simulink model "ModelMotS_AlphaBeta_bis_FVC"  (R2018b)
settings: Solver=ode45  StartTime=0.0  StopTime=1200  MaxStep=1e-4  RelTol=1e-4  EnableMultiTasking=on
values from neighbouring files (symbols this model uses):
  Data_Ts = 0.005    [gen_sim_alpha_beta.m]    (also in gen_sim_dq.m = 0.00025)
  Inom = 9.1    [gen_sim_alpha_beta.m]    (also in gen_sim_dq.m)
  J = 0.045    [gen_sim_alpha_beta.m]    (also in gen_sim_dq.m; gen_sim_new_data_december.m)
  Jm = J    (= 0.045)    [gen_sim_alpha_beta.m]    (also in gen_sim_dq.m)
  Lfr = 0.007    [gen_sim_alpha_beta.m]    (also in gen_sim_dq.m; gen_sim_new_data_december.m)
  Lfs = 0.007    [gen_sim_alpha_beta.m]    (also in gen_sim_dq.m; gen_sim_new_data_december.m)
  Lm = 0.153    [gen_sim_alpha_beta.m]    (also in gen_sim_dq.m; gen_sim_new_data_december.m)
  Lmt = 0.210    (= 0.21)    [gen_sim_alpha_beta.m]    (also in gen_sim_dq.m; gen_sim_new_data_december.m)
  Lr = 0.160    (= 0.16)    [gen_sim_alpha_beta.m]    (also in gen_sim_dq.m; gen_sim_new_data_december.m)
  Ls = 0.160    (= 0.16)    [gen_sim_alpha_beta.m]    (also in gen_sim_dq.m; gen_sim_new_data_december.m)
  np = 2    [gen_sim_alpha_beta.m]    (also in gen_sim_dq.m; gen_sim_new_data_december.m)
  P1 = 0.7    [gen_sim_alpha_beta.m]    (also in gen_sim_dq.m; gen_sim_new_data_december.m)
  P2 = 1.5    [gen_sim_alpha_beta.m]    (also in gen_sim_dq.m; gen_sim_new_data_december.m)
  Prdnom = 1    [gen_sim_alpha_beta.m]    (also in gen_sim_dq.m)
  Prinit = [ 0 ; 0 ]    [gen_sim_alpha_beta.m]    (also in gen_sim_dq.m; gen_sim_new_data_december.m)
  Psinit = [ 0 ; 0 ]    [gen_sim_alpha_beta.m]    (also in gen_sim_dq.m; gen_sim_new_data_december.m)
  Rr = 0.9    [gen_sim_alpha_beta.m]    (also in gen_sim_dq.m; gen_sim_new_data_december.m)
  Rs = 1.5    [gen_sim_alpha_beta.m]    (also in gen_sim_dq.m; gen_sim_new_data_december.m)
  SFC_Coeff = 100    [gen_sim_alpha_beta.m]    (also in gen_sim_dq.m)
  SLP_Coeff = 100    [gen_sim_alpha_beta.m]    (also in gen_sim_dq.m)
  Speed = data.speed_true    [Plot_EncoderDecoder_Output.m]    (also in TreatModelMot_dq.m = Data.Speed.Data / (2*pi); test1.mat = [0 0 0 0 0 0 0 0 0 0 0 0 ... (601 elements, 601x1)]; test2.mat = [0 0 0 0 0 0 0 0 0 0 0 0 ... (601 elements, 601x1)])
  thrinit = 0    [gen_sim_alpha_beta.m]    (also in gen_sim_dq.m; gen_sim_new_data_december.m)
  Tn = 25    [gen_sim_alpha_beta.m]    (also in gen_sim_dq.m; gen_sim_new_data_december.m)
  Tpwm = Ts    (= 0.00025)    [gen_sim_alpha_beta.m]    (also in gen_sim_dq.m)
  Vnom = 400    [gen_sim_alpha_beta.m]    (also in gen_sim_dq.m)
  wCurr = 0    [gen_sim_alpha_beta.m]    (also in gen_sim_dq.m)
  wCurr_PI = 2*pi*50    (= 314.159265359)    [gen_sim_alpha_beta.m]    (also in gen_sim_dq.m)
  wL = 2*pi*0    (= 0)    [gen_sim_alpha_beta.m]    (also in gen_sim_dq.m; gen_sim_new_data_december.m)
  wn = 2*pi*50    (= 314.159265359)    [gen_sim_alpha_beta.m]    (also in gen_sim_dq.m; gen_sim_new_data_december.m)
  wrinit = 2*pi*0    (= 0)    [gen_sim_alpha_beta.m]    (also in gen_sim_dq.m; gen_sim_new_data_december.m)
  wSpeed_PI = 2*pi*2.5    (= 15.7079632679)    [gen_sim_alpha_beta.m]    (also in gen_sim_dq.m)
  wSpeedEst = 2*pi*500    (= 3141.59265359)    [gen_sim_alpha_beta.m]    (also in gen_sim_dq.m)
  xiCurr_PI = 1/2    (= 0.5)    [gen_sim_alpha_beta.m]    (also in gen_sim_dq.m)
  xiSpeed_PI = 1    [gen_sim_alpha_beta.m]    (also in gen_sim_dq.m)
undefined symbols (not defined in the file or in its folder): DiscIntNeverNeededParam, TorqueLoad
libraries: simulink x7
settings Model: Creator=stbp106  LastModifiedBy=SESA336393
settings DataIOCC: LimitDataPoints=on  SaveFormat=Array
settings OptimizationCC: LifeSpan=inf
settings DebuggingCC: UnderspecifiedInitializationDetection=Classic  MergeDetectMultiDrivingBlocksExec=none  SolverPrmCheckMsg=warning  SFUnexpectedBacktrackingDiag=warning  SFNoUnconditionalDefaultTransitionDiag=warning  SFExecutionAtInitializationDiag=none
settings HardwareCC: ProdBitPerPointer=32  ProdBitPerSizeT=32  ProdBitPerPtrDiffT=32  ProdLargestAtomicFloat=None  ProdIntDivRoundTo=Undefined  ProdEndianess=Unspecified  ProdWordSize=32  ProdHWDeviceType=32-bit Generic
settings ModelReferenceCC: PropagateSignalLabelsOutOfModel=off
settings SFSimCC: SimUseLocalCustomCode=off
settings RTWCC: RTWUseLocalCustomCode=off
settings CodeAppCC: StateflowObjectComments=on
settings GRTTargetCC: TargetLangStandard=C89/C90 (ANSI)  GeneratePreprocessorConditionals=Disable all
settings ConfigComp: CovMetricSettings=dw  CovHtmlReporting=on  CovSaveCumulativeToWorkspaceVar=on  CovSaveSingleToWorkspaceVar=on  CovExternalEMLEnable=off  CovSFcnEnable=off

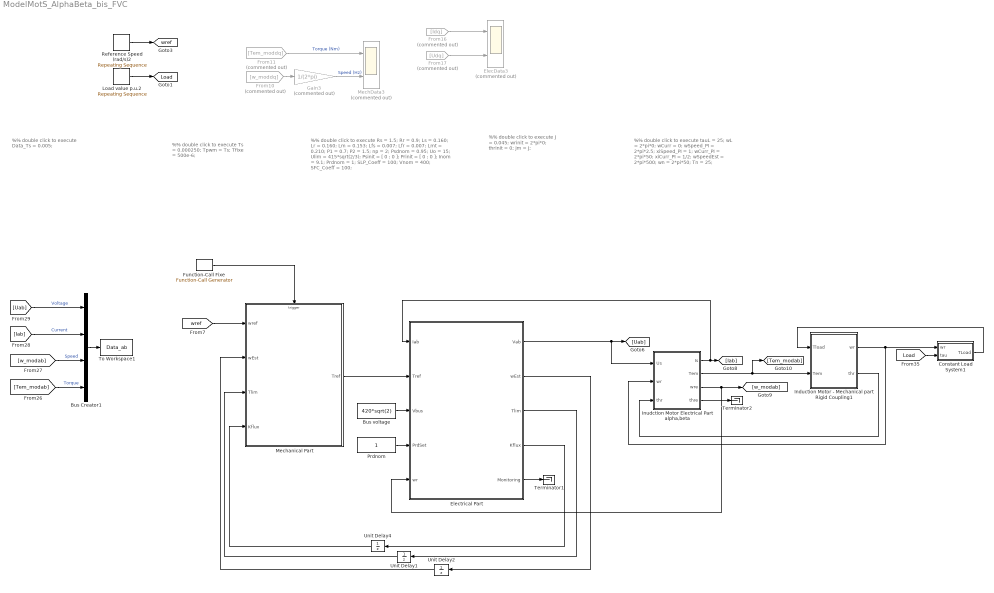
== system ModelMotS_AlphaBeta_bis_FVC ==
  note: %% double click to execute
      |
      | Rs = 1.5; Rr = 0.9;
      | Ls = 0.160; Lr = 0.160; Lm = 0.153;
      | Lfs = 0.007; Lfr = 0.007; Lmt = 0.210; P1 = 0.7; P2 = 1.5;
      | np = 2;
      | Psdnom = 0.95; Uo = 15; Ulim = 415*sqrt(2/3);
      | Psinit = [ 0 ; 0 ]; Prinit = [ 0 ; 0 ];
      | Inom = 9.1; Prdnom = 1; SLP_Coeff = 100; Vnom = 400;
      | SFC_Coeff = 100;
  note: %% double click to execute
      |
      | J = 0.045;
      | wrinit = 2*pi*0;
      | thrinit = 0;
      | Jm = J;
  note: %% double click to execute
      |
      | tauL = 25;
      | wL = 2*pi*0;
      |
      | wCurr = 0;
      | wSpeed_PI = 2*pi*2.5; xiSpeed_PI = 1;
      | wCurr_PI = 2*pi*50; xiCurr_PI = 1/2;
      | wSpeedEst = 2*pi*500;
      |
      | wn = 2*pi*50;
      | Tn = 25;
  note: %% double click to execute
      |
      | Ts = 0.000250;
      | Tpwm = Ts;
      | Tfixe = 500e-6;
  note: %% double click to execute
      |
      | Data_Ts = 0.005;
  Bus Creator1 : BusCreator  Inputs=4
  Bus voltage : Constant  Value=420*sqrt(2)
  Constant Load System1 : Subsystem  Description=""
  ElecData3 : Scope  Commented=on  NumInputPorts=2
  Electrical Part : Subsystem
  From10 : From  Commented=on  GotoTag=w_moddq
  From11 : From  Commented=on  GotoTag=Tem_moddq
  From16 : From  Commented=on  GotoTag=Idq
  From17 : From  Commented=on  GotoTag=Udq
  Function-Call Fixe : simulink/Ports & Subsystems/Function-Call Generator  sample_time=Tfixe  numberOfIterations=1
  Gain3 : Gain  Commented=on  Gain=1/(2*pi)  SaturateOnIntegerOverflow=on  OutDataTypeStr=Inherit: Same as input  ParamDataTypeStr=Inherit: Same as input
  Induction Motor - Mechanical part Rigid Coupling1 : Subsystem  Description=""
  Inudction Motor Electrical Part alpha,beta : Subsystem  Description=""
  Load value p.u.2 : simulink/Sources/Repeating Sequence  rep_seq_t=t  rep_seq_y=TorqueLoad*Tn
  MechData3 : Scope  Commented=on  NumInputPorts=2
  Mechanical Part : Subsystem
  Prdnom : Constant
  Reference Speed (rad/s)2 : simulink/Sources/Repeating Sequence  rep_seq_t=t  rep_seq_y=Speed*wn
  Terminator1 : Terminator
  Terminator2 : Terminator
  To Workspace1 : ToWorkspace  VariableName=Data_ab  SaveFormat=Timeseries  SampleTime=Data_Ts
  Unit Delay1 : UnitDelay  SampleTime=-1
  Unit Delay2 : UnitDelay  SampleTime=-1
  Unit Delay4 : UnitDelay  SampleTime=-1
  tag scope: Load=global, wref=global
  wires:
  From16/1 -> ElecData3/1
  From17/1 -> ElecData3/2
  From10/1 -> Gain3/1
  From11/1 -> MechData3/1  "Torque (Nm)"
  Gain3/1 -> MechData3/2  "Speed (Hz)"
  Induction Motor - Mechanical part Rigid Coupling1/2(thr) -> Inudction Motor Electrical Part alpha,beta/3(thr)
  Inudction Motor Electrical Part alpha,beta/2(Tem) -> [Tem_modab], Induction Motor - Mechanical part Rigid Coupling1/2(Tem)
  Induction Motor - Mechanical part Rigid Coupling1/1(wr) -> Constant Load System1/1(wr), Inudction Motor Electrical Part alpha,beta/2(wr)
  Inudction Motor Electrical Part alpha,beta/4(thre) -> Terminator2/1
  Constant Load System1/1(TLoad) -> Induction Motor - Mechanical part Rigid Coupling1/1(Tload)
  [Load] -> Constant Load System1/2(tau)
  Electrical Part/1(Vab) -> Inudction Motor Electrical Part alpha,beta/1(Us), [Uab]
  Reference Speed (rad/s)2/1 -> [wref]
  Load value p.u.2/1 -> [Load]
  Prdnom/1 -> Electrical Part/4(PrdSet)
  Inudction Motor Electrical Part alpha,beta/3(wre) -> Electrical Part/5(wr), [w_modab]
  Electrical Part/3(Tlim) -> Unit Delay1/1
  Electrical Part/4(Kflux) -> Unit Delay4/1
  Unit Delay1/1 -> Mechanical Part/3(Tlim)
  [wref] -> Mechanical Part/1(wref)
  Unit Delay4/1 -> Mechanical Part/4(Kflux)
  Bus voltage/1 -> Electrical Part/3(Vbus)
  Unit Delay2/1 -> Mechanical Part/2(wEst)
  Mechanical Part/1(Tref) -> Electrical Part/2(Tref)
  Inudction Motor Electrical Part alpha,beta/1(Is) -> Electrical Part/1(Iab), [Iab]
  Function-Call Fixe/1 -> Mechanical Part/Trigger
  Electrical Part/2(wEst) -> Unit Delay2/1
  Electrical Part/5(Monitoring) -> Terminator1/1
  Bus Creator1/1 -> To Workspace1/1
  [w_modab] -> Bus Creator1/3  "Speed"
  [Tem_modab] -> Bus Creator1/4  "Torque"
  [Iab] -> Bus Creator1/2  "Current"
  [Uab] -> Bus Creator1/1  "Voltage"

== system ModelMotS_AlphaBeta_bis_FVC/Constant Load System1 ==
  wr : Inport
  tau : Inport  Port=2
  Constant1 : Constant  Value=wL
  Fcn : Fcn  Expr=u(1)/sqrt( u(1)^2 + (2*pi*0.1)^2)
  Product2 : Product  RndMeth=Zero
  Sum2 : Sum  Inputs=+-  SaturateOnIntegerOverflow=on  InputSameDT=on  OutDataTypeStr=Inherit: Same as first input
  TLoad : Outport
  wires:
  Product2/1 -> TLoad/1
  wr/1 -> Sum2/1
  Constant1/1 -> Sum2/2
  Sum2/1 -> Fcn/1
  Fcn/1 -> Product2/1
  tau/1 -> Product2/2

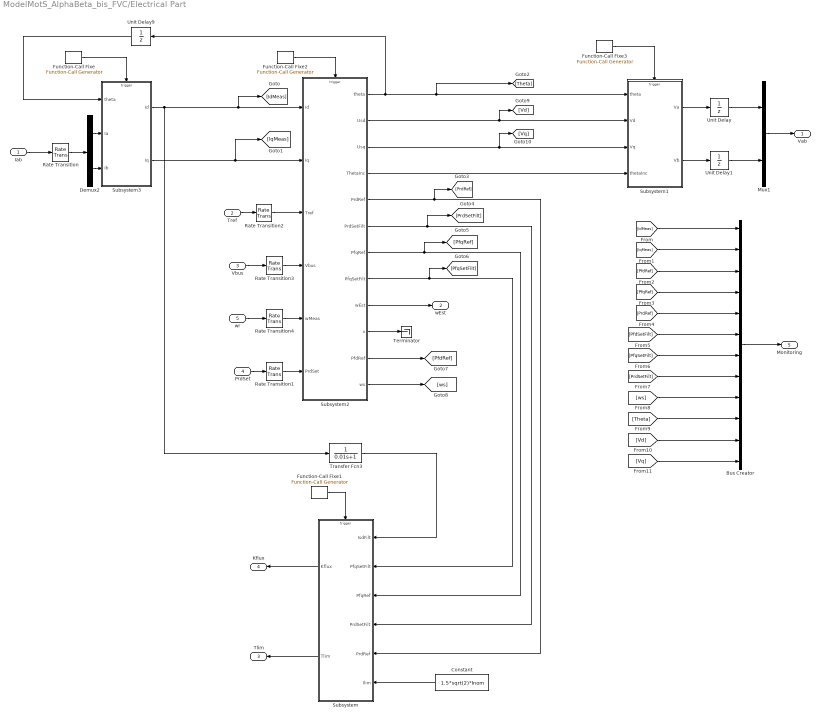
== system ModelMotS_AlphaBeta_bis_FVC/Electrical Part ==
  Iab : Inport
  Tref : Inport  Port=2
  Vbus : Inport  Port=3
  PrdSet : Inport  Port=4
  wr : Inport  Port=5
  Bus Creator : BusCreator  Inputs=12
  Constant : Constant  Value=1.5*sqrt(2)*Inom
  Demux2 : Demux  Outputs=2
  Function-Call Fixe : simulink/Ports & Subsystems/Function-Call Generator  sample_time=Tpwm  numberOfIterations=1
  Function-Call Fixe1 : simulink/Ports & Subsystems/Function-Call Generator  sample_time=Tfixe  numberOfIterations=1
  Function-Call Fixe2 : simulink/Ports & Subsystems/Function-Call Generator  sample_time=Tpwm  numberOfIterations=1
  Function-Call Fixe3 : simulink/Ports & Subsystems/Function-Call Generator  sample_time=Tpwm  numberOfIterations=1
  Mux1 : Mux  Inputs=2
  Rate Transition{,1..4} (5 alike) : RateTransition
  Subsystem : Subsystem
  Subsystem1 : Subsystem
  Subsystem2 : Subsystem
  Subsystem3 : Subsystem
  Terminator : Terminator
  Transfer Fcn3 : TransferFcn  Denominator=[0.01 1]
  Unit Delay : UnitDelay  SampleTime=-1
  Unit Delay1 : UnitDelay  SampleTime=-1
  Unit Delay9 : UnitDelay  SampleTime=-1
  Vab : Outport
  wEst : Outport  Port=2
  Tlim : Outport  Port=3
  Kflux : Outport  Port=4
  Monitoring : Outport  Port=5
  wires:
  [IqMeas] -> Bus Creator/2
  [IdMeas] -> Bus Creator/1
  [PfdRef] -> Bus Creator/3
  [PfqRef] -> Bus Creator/4
  [PrdRef] -> Bus Creator/5
  [PrdSetFilt] -> Bus Creator/8
  [PfqSetFilt] -> Bus Creator/7
  [PfdSetFilt] -> Bus Creator/6
  [ws] -> Bus Creator/9
  [Theta] -> Bus Creator/10
  Bus Creator/1 -> Monitoring/1
  Transfer Fcn3/1 -> Subsystem/1(IsdFilt)
  Subsystem/1(Kflux) -> Kflux/1
  Subsystem/2(Tlim) -> Tlim/1
  Subsystem1/1(Va) -> Unit Delay/1
  [Vd] -> Bus Creator/11
  [Vq] -> Bus Creator/12
  Subsystem2/7(PfqRef) -> [PfqRef], Subsystem/3(PfqRef)
  Subsystem2/6(PrdSetFilt) -> [PrdSetFilt], Subsystem/4(PrdSetFilt)
  Subsystem2/8(PfqSetFilt) -> [PfqSetFilt], Subsystem/2(PfqSetFilt)
  Subsystem2/1(theta) -> Subsystem1/1(theta), [Theta], Unit Delay9/1
  Subsystem2/5(PrdRef) -> [PrdRef], Subsystem/5(PrdRef)
  Subsystem2/3(Usq) -> [Vq], Subsystem1/3(Vq)
  Subsystem2/2(Usd) -> Subsystem1/2(Vd), [Vd]
  Tref/1 -> Rate Transition2/1
  Vbus/1 -> Rate Transition3/1
  wr/1 -> Rate Transition4/1
  Subsystem2/4(ThetaInc) -> Subsystem1/4(thetaInc)
  Subsystem2/9(wEst) -> wEst/1
  Subsystem2/11(PfdRef) -> [PfdRef]
  Subsystem2/12(ws) -> [ws]
  Subsystem3/2(Iq) -> [IqMeas], Subsystem2/2(Iq)
  Subsystem3/1(Id) -> Transfer Fcn3/1, Subsystem2/1(Id), [IdMeas]
  Unit Delay9/1 -> Subsystem3/1(theta)
  Iab/1 -> Rate Transition/1
  Function-Call Fixe/1 -> Subsystem3/Trigger
  Function-Call Fixe2/1 -> Subsystem2/Trigger
  Function-Call Fixe3/1 -> Subsystem1/Trigger
  Function-Call Fixe1/1 -> Subsystem/Trigger
  Rate Transition2/1 -> Subsystem2/3(Tref)
  Subsystem2/10(x) -> Terminator/1
  Constant/1 -> Subsystem/6(Ilim)
  Rate Transition3/1 -> Subsystem2/4(Vbus)
  Rate Transition4/1 -> Subsystem2/5(wMeas)
  Rate Transition/1 -> Demux2/1
  Demux2/1 -> Subsystem3/2(Ia)
  Demux2/2 -> Subsystem3/3(Ib)
  Subsystem1/2(Vb) -> Unit Delay1/1
  Unit Delay/1 -> Mux1/1
  Unit Delay1/1 -> Mux1/2
  Mux1/1 -> Vab/1
  PrdSet/1 -> Rate Transition1/1
  Rate Transition1/1 -> Subsystem2/6(PrdSet)

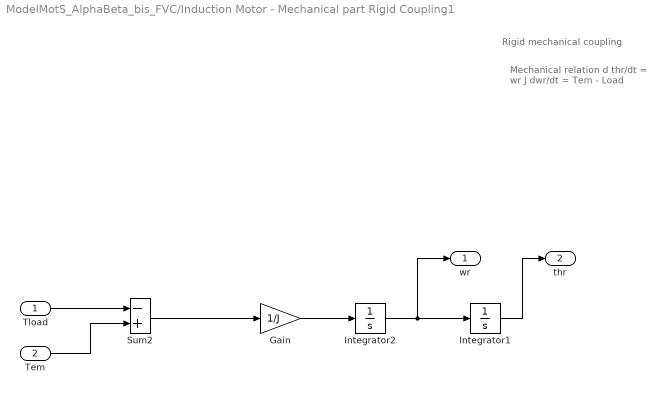
== system ModelMotS_AlphaBeta_bis_FVC/Induction Motor - Mechanical part Rigid Coupling1 ==
  note: Mechanical relation
      | d thr/dt = wr
      | J dwr/dt = Tem - Load
  note: Rigid mechanical coupling
  Tload : Inport
  Tem : Inport  Port=2
  Gain : Gain  Gain=1/J  SaturateOnIntegerOverflow=on  OutDataTypeStr=Inherit: Same as input  ParamDataTypeStr=Inherit: Same as input
  Integrator1 : Integrator  InitialCondition=thrinit
  Integrator2 : Integrator  InitialCondition=wrinit
  Sum2 : Sum  Inputs=-+  SaturateOnIntegerOverflow=on  InputSameDT=on  OutDataTypeStr=Inherit: Same as first input
  wr : Outport
  thr : Outport  Port=2
  wires:
  Sum2/1 -> Gain/1
  Gain/1 -> Integrator2/1
  Tload/1 -> Sum2/1
  Tem/1 -> Sum2/2
  Integrator2/1 -> Integrator1/1, wr/1
  Integrator1/1 -> thr/1

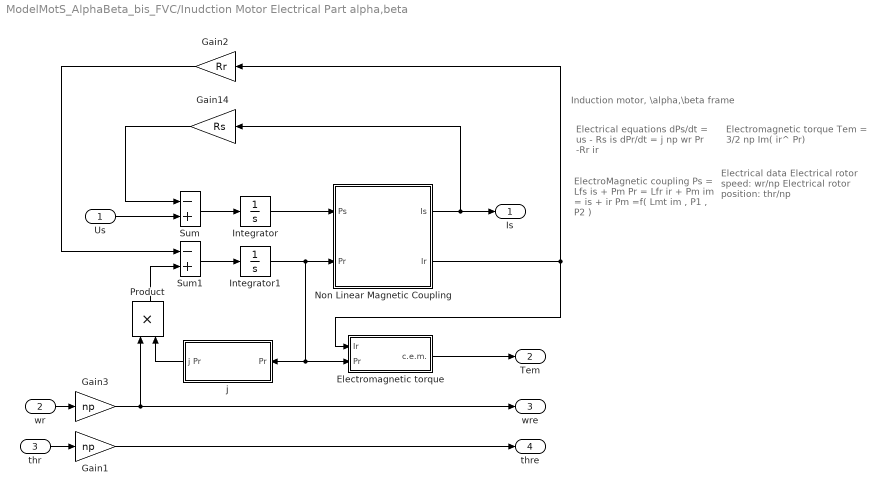
== system ModelMotS_AlphaBeta_bis_FVC/Inudction Motor Electrical Part alpha,beta ==
  note: Electrical equations
      | dPs/dt = us - Rs is
      | dPr/dt = j np wr Pr -Rr ir
  note: ElectroMagnetic coupling
      | Ps  = Lfs is + Pm
      | Pr  = Lfr ir + Pm
      |
      | im = is + ir
      | Pm =f( Lmt im , P1 , P2 )
  note: Electromagnetic torque
      | Tem = 3/2 np Im( ir^ Pr)
  note: Induction motor, \alpha,\beta frame
  note: Electrical data
      | Electrical rotor speed: wr/np
      | Electrical rotor position: thr/np
  Us : Inport
  wr : Inport  Port=2
  thr : Inport  Port=3
  Electromagnetic torque : Subsystem
  Gain1 : Gain  Gain=np  SaturateOnIntegerOverflow=on  OutDataTypeStr=Inherit: Same as input  ParamDataTypeStr=Inherit: Same as input
  Gain14 : Gain  Gain=Rs  SaturateOnIntegerOverflow=on  OutDataTypeStr=Inherit: Same as input  ParamDataTypeStr=Inherit: Same as input
  Gain2 : Gain  Gain=Rr  SaturateOnIntegerOverflow=on  OutDataTypeStr=Inherit: Same as input  ParamDataTypeStr=Inherit: Same as input
  Gain3 : Gain  Gain=np  SaturateOnIntegerOverflow=on  OutDataTypeStr=Inherit: Same as input  ParamDataTypeStr=Inherit: Same as input
  Integrator : Integrator  InitialCondition=Psinit
  Integrator1 : Integrator  InitialCondition=Prinit
  Non Linear Magnetic Coupling : Subsystem
  Product : Product  SaturateOnIntegerOverflow=on  RndMeth=Zero  InputSameDT=on  OutDataTypeStr=Inherit: Same as first input
  Sum : Sum  Inputs=-+  SaturateOnIntegerOverflow=on  InputSameDT=on  OutDataTypeStr=Inherit: Same as first input
  Sum1 : Sum  Inputs=-+  SaturateOnIntegerOverflow=on  InputSameDT=on  OutDataTypeStr=Inherit: Same as first input
  j : Subsystem
  Is : Outport
  Tem : Outport  Port=2
  wre : Outport  Port=3
  thre : Outport  Port=4
  wires:
  Sum/1 -> Integrator/1
  Non Linear Magnetic Coupling/1(Is) -> Gain14/1, Is/1
  Gain14/1 -> Sum/1
  Us/1 -> Sum/2
  Sum1/1 -> Integrator1/1
  Gain2/1 -> Sum1/1
  j/1(j Pr) -> Product/2
  Product/1 -> Sum1/2
  Non Linear Magnetic Coupling/2(Ir) -> Electromagnetic torque/1(Ir), Gain2/1
  Electromagnetic torque/1(c.e.m.) -> Tem/1
  Integrator/1 -> Non Linear Magnetic Coupling/1(Ps)
  Integrator1/1 -> Non Linear Magnetic Coupling/2(Pr), j/1(Pr), Electromagnetic torque/2(Pr)
  Gain3/1 -> Product/1, wre/1
  wr/1 -> Gain3/1
  thr/1 -> Gain1/1
  Gain1/1 -> thre/1

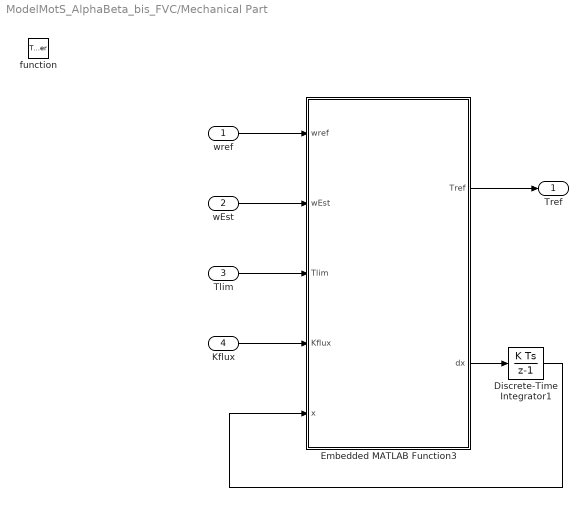
== system ModelMotS_AlphaBeta_bis_FVC/Mechanical Part ==
  wref : Inport
  wEst : Inport  Port=2
  Tlim : Inport  Port=3
  Kflux : Inport  Port=4
  function : TriggerPort  TriggerType=function-call  VariantControl=(inherit)
  Discrete-Time Integrator1 : DiscreteIntegrator  InitialCondition=zeros(1,2)  SampleTime=-1  ICPrevOutput=DiscIntNeverNeededParam  ICPrevScaledInput=DiscIntNeverNeededParam
  Embedded MATLAB Function3 : MATLAB Function  TreatAsAtomicUnit=on
  Tref : Outport
  wires:
  Discrete-Time Integrator1/1 -> Embedded MATLAB Function3/5(x)
  wEst/1 -> Embedded MATLAB Function3/2(wEst)
  Tlim/1 -> Embedded MATLAB Function3/3(Tlim)
  wref/1 -> Embedded MATLAB Function3/1(wref)
  Embedded MATLAB Function3/2(dx) -> Discrete-Time Integrator1/1
  Embedded MATLAB Function3/1(Tref) -> Tref/1
  Kflux/1 -> Embedded MATLAB Function3/4(Kflux)

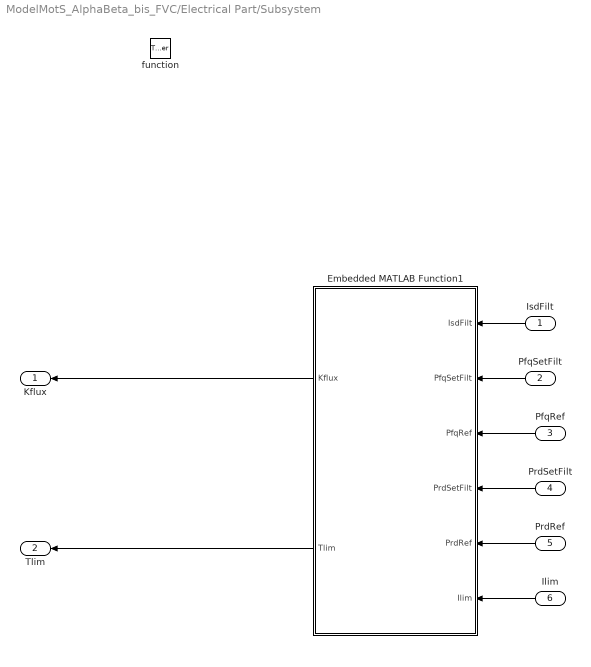
== system ModelMotS_AlphaBeta_bis_FVC/Electrical Part/Subsystem ==
  IsdFilt : Inport
  PfqSetFilt : Inport  Port=2
  PfqRef : Inport  Port=3
  PrdSetFilt : Inport  Port=4
  PrdRef : Inport  Port=5
  Ilim : Inport  Port=6
  function : TriggerPort  TriggerType=function-call  VariantControl=(inherit)
  Embedded MATLAB Function1 : MATLAB Function  TreatAsAtomicUnit=on
  Kflux : Outport
  Tlim : Outport  Port=2
  wires:
  Embedded MATLAB Function1/2(Tlim) -> Tlim/1
  IsdFilt/1 -> Embedded MATLAB Function1/1(IsdFilt)
  Embedded MATLAB Function1/1(Kflux) -> Kflux/1
  PrdSetFilt/1 -> Embedded MATLAB Function1/4(PrdSetFilt)
  PfqSetFilt/1 -> Embedded MATLAB Function1/2(PfqSetFilt)
  PfqRef/1 -> Embedded MATLAB Function1/3(PfqRef)
  PrdRef/1 -> Embedded MATLAB Function1/5(PrdRef)
  Ilim/1 -> Embedded MATLAB Function1/6(Ilim)

== system ModelMotS_AlphaBeta_bis_FVC/Electrical Part/Subsystem1 ==
  theta : Inport
  Vd : Inport  Port=2
  Vq : Inport  Port=3
  thetaInc : Inport  Port=4
  function : TriggerPort  TriggerType=function-call  VariantControl=(inherit)
  Embedded MATLAB Function5 : MATLAB Function  TreatAsAtomicUnit=on
  Va : Outport
  Vb : Outport  Port=2
  wires:
  Embedded MATLAB Function5/1(Va) -> Va/1
  Vd/1 -> Embedded MATLAB Function5/1(Vd)
  thetaInc/1 -> Embedded MATLAB Function5/4(thetaInc)
  Embedded MATLAB Function5/2(Vb) -> Vb/1
  Vq/1 -> Embedded MATLAB Function5/2(Vq)
  theta/1 -> Embedded MATLAB Function5/3(theta)

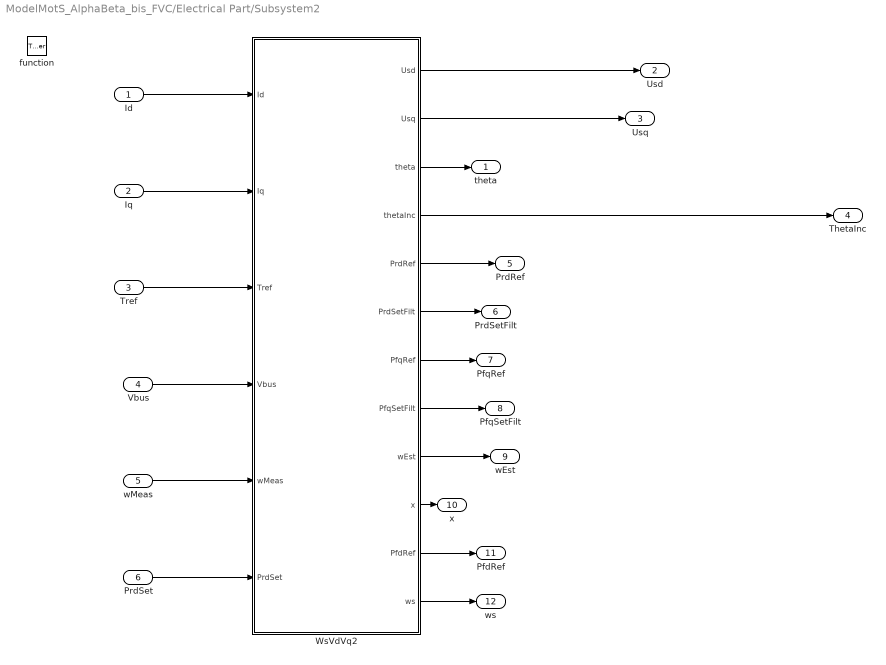
== system ModelMotS_AlphaBeta_bis_FVC/Electrical Part/Subsystem2 ==
  Id : Inport
  Iq : Inport  Port=2
  Tref : Inport  Port=3
  Vbus : Inport  Port=4
  wMeas : Inport  Port=5
  PrdSet : Inport  Port=6
  function : TriggerPort  TriggerType=function-call  VariantControl=(inherit)
  WsVdVq2 : Subsystem
  theta : Outport
  Usd : Outport  Port=2
  Usq : Outport  Port=3
  ThetaInc : Outport  Port=4
  PrdRef : Outport  Port=5
  PrdSetFilt : Outport  Port=6
  PfqRef : Outport  Port=7
  PfqSetFilt : Outport  Port=8
  wEst : Outport  Port=9
  x : Outport  Port=10
  PfdRef : Outport  Port=11
  ws : Outport  Port=12
  wires:
  WsVdVq2/7(PfqRef) -> PfqRef/1
  WsVdVq2/9(wEst) -> wEst/1
  Tref/1 -> WsVdVq2/3(Tref)
  WsVdVq2/8(PfqSetFilt) -> PfqSetFilt/1
  WsVdVq2/6(PrdSetFilt) -> PrdSetFilt/1
  Vbus/1 -> WsVdVq2/4(Vbus)
  wMeas/1 -> WsVdVq2/5(wMeas)
  WsVdVq2/5(PrdRef) -> PrdRef/1
  WsVdVq2/3(theta) -> theta/1
  WsVdVq2/12(ws) -> ws/1
  WsVdVq2/11(PfdRef) -> PfdRef/1
  WsVdVq2/2(Usq) -> Usq/1
  WsVdVq2/4(thetaInc) -> ThetaInc/1
  WsVdVq2/1(Usd) -> Usd/1
  WsVdVq2/10(x) -> x/1
  Id/1 -> WsVdVq2/1(Id)
  Iq/1 -> WsVdVq2/2(Iq)
  PrdSet/1 -> WsVdVq2/6(PrdSet)

== system ModelMotS_AlphaBeta_bis_FVC/Electrical Part/Subsystem3 ==
  theta : Inport
  Ia : Inport  Port=2
  Ib : Inport  Port=3
  function : TriggerPort  TriggerType=function-call  VariantControl=(inherit)
  Embedded MATLAB Function2 : MATLAB Function  TreatAsAtomicUnit=on
  Id : Outport
  Iq : Outport  Port=2
  wires:
  Embedded MATLAB Function2/1(Id) -> Id/1
  Ia/1 -> Embedded MATLAB Function2/1(Ia)
  theta/1 -> Embedded MATLAB Function2/3(theta)
  Ib/1 -> Embedded MATLAB Function2/2(Ib)
  Embedded MATLAB Function2/2(Iq) -> Iq/1

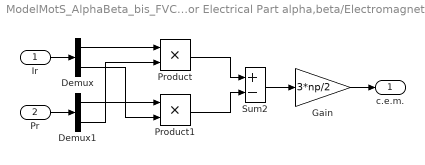
== system ModelMotS_AlphaBeta_bis_FVC/Inudction Motor Electrical Part alpha,beta/Electromagnetic torque ==
  Ir : Inport
  Pr : Inport  Port=2
  Demux : Demux  Outputs=2
  Demux1 : Demux  Outputs=2
  Gain : Gain  Gain=3*np/2  SaturateOnIntegerOverflow=on  OutDataTypeStr=Inherit: Same as input  ParamDataTypeStr=Inherit: Same as input
  Product : Product  SaturateOnIntegerOverflow=on  RndMeth=Zero  InputSameDT=on  OutDataTypeStr=Inherit: Same as first input
  Product1 : Product  SaturateOnIntegerOverflow=on  RndMeth=Zero  InputSameDT=on  OutDataTypeStr=Inherit: Same as first input
  Sum2 : Sum  Inputs=+-  SaturateOnIntegerOverflow=on  InputSameDT=on  OutDataTypeStr=Inherit: Same as first input
  c.e.m. : Outport
  wires:
  Product/1 -> Sum2/1
  Product1/1 -> Sum2/2
  Sum2/1 -> Gain/1
  Demux/1 -> Product/1
  Demux1/2 -> Product/2
  Demux1/1 -> Product1/1
  Demux/2 -> Product1/2
  Ir/1 -> Demux/1
  Gain/1 -> c.e.m./1
  Pr/1 -> Demux1/1

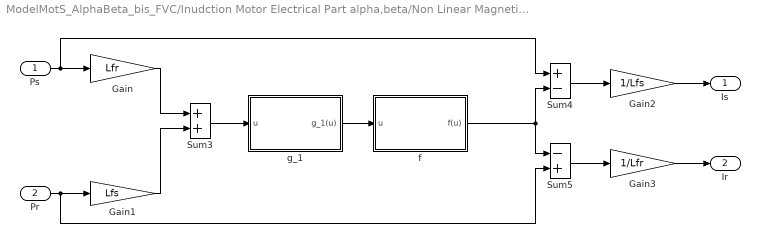
== system ModelMotS_AlphaBeta_bis_FVC/Inudction Motor Electrical Part alpha,beta/Non Linear Magnetic Coupling ==
  Ps : Inport
  Pr : Inport  Port=2
  Gain : Gain  Gain=Lfr  SaturateOnIntegerOverflow=on  OutDataTypeStr=Inherit: Same as input  ParamDataTypeStr=Inherit: Same as input
  Gain1 : Gain  Gain=Lfs  SaturateOnIntegerOverflow=on  OutDataTypeStr=Inherit: Same as input  ParamDataTypeStr=Inherit: Same as input
  Gain2 : Gain  Gain=1/Lfs  SaturateOnIntegerOverflow=on  OutDataTypeStr=Inherit: Same as input  ParamDataTypeStr=Inherit: Same as input
  Gain3 : Gain  Gain=1/Lfr  SaturateOnIntegerOverflow=on  OutDataTypeStr=Inherit: Same as input  ParamDataTypeStr=Inherit: Same as input
  Sum3 : Sum  SaturateOnIntegerOverflow=on  InputSameDT=on  OutDataTypeStr=Inherit: Same as first input
  Sum4 : Sum  Inputs=+-  SaturateOnIntegerOverflow=on  InputSameDT=on  OutDataTypeStr=Inherit: Same as first input
  Sum5 : Sum  Inputs=-+  SaturateOnIntegerOverflow=on  InputSameDT=on  OutDataTypeStr=Inherit: Same as first input
  f : Subsystem
  g_1 : Subsystem
  Is : Outport
  Ir : Outport  Port=2
  wires:
  Gain2/1 -> Is/1
  Gain3/1 -> Ir/1
  Sum5/1 -> Gain3/1
  Sum4/1 -> Gain2/1
  Pr/1 -> Sum5/2, Gain1/1
  Ps/1 -> Sum4/1, Gain/1
  f/1(f(u)) -> Sum4/2, Sum5/1
  g_1/1(g_1(u)) -> f/1(u)
  Sum3/1 -> g_1/1(u)
  Gain1/1 -> Sum3/2
  Gain/1 -> Sum3/1

== system ModelMotS_AlphaBeta_bis_FVC/Inudction Motor Electrical Part alpha,beta/j ==
  Pr : Inport
  Demux1 : Demux  Outputs=2
  Gain : Gain  Gain=-1  SaturateOnIntegerOverflow=on  OutDataTypeStr=Inherit: Same as input  ParamDataTypeStr=Inherit: Same as input
  Mux : Mux  Inputs=2
  j Pr : Outport
  wires:
  Pr/1 -> Demux1/1
  Demux1/1 -> Mux/2
  Demux1/2 -> Gain/1
  Gain/1 -> Mux/1
  Mux/1 -> j Pr/1

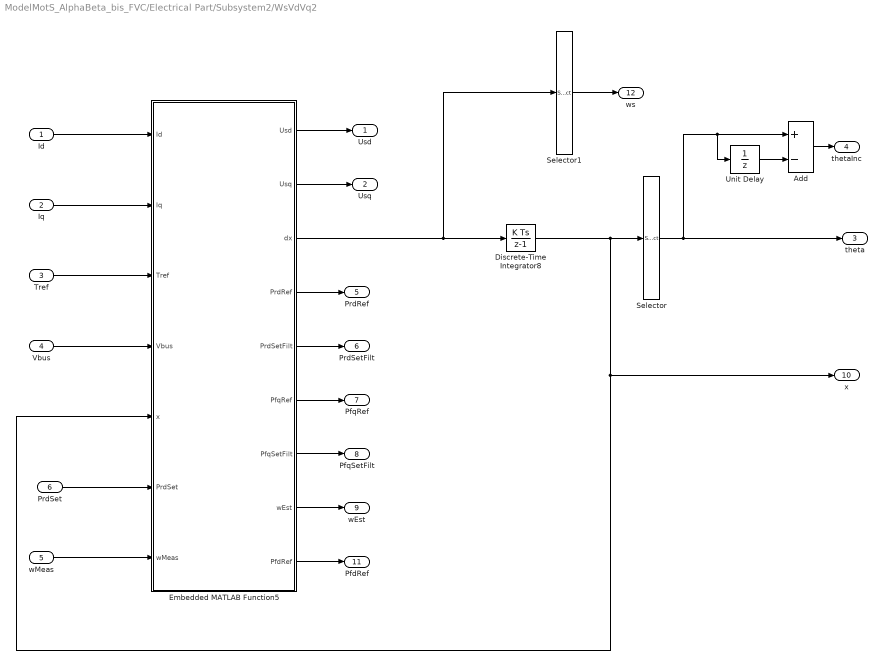
== system ModelMotS_AlphaBeta_bis_FVC/Electrical Part/Subsystem2/WsVdVq2 ==
  Id : Inport
  Iq : Inport  Port=2
  Tref : Inport  Port=3
  Vbus : Inport  Port=4
  wMeas : Inport  Port=5
  PrdSet : Inport  Port=6
  Add : Sum  Inputs=+-
  Discrete-Time Integrator8 : DiscreteIntegrator  InitialCondition=zeros(1,12)  SampleTime=-1  ICPrevOutput=DiscIntNeverNeededParam  ICPrevScaledInput=DiscIntNeverNeededParam
  Embedded MATLAB Function5 : MATLAB Function  TreatAsAtomicUnit=on
  Selector : Selector  InputPortWidth=12  IndexOptions=Index vector (dialog)  Indices=5  OutputSizes=1
  Selector1 : Selector  InputPortWidth=12  IndexOptions=Index vector (dialog)  Indices=5  OutputSizes=1
  Unit Delay : UnitDelay  SampleTime=-1
  Usd : Outport
  Usq : Outport  Port=2
  theta : Outport  Port=3  InitialOutput=[0]
  thetaInc : Outport  Port=4  InitialOutput=[0]
  PrdRef : Outport  Port=5
  PrdSetFilt : Outport  Port=6
  PfqRef : Outport  Port=7
  PfqSetFilt : Outport  Port=8
  wEst : Outport  Port=9
  x : Outport  Port=10  InitialOutput=[0]
  PfdRef : Outport  Port=11
  ws : Outport  Port=12  InitialOutput=[0]
  wires:
  wMeas/1 -> Embedded MATLAB Function5/7(wMeas)
  Unit Delay/1 -> Add/2
  Selector/1 -> theta/1, Unit Delay/1, Add/1
  Add/1 -> thetaInc/1
  Embedded MATLAB Function5/7(PfqSetFilt) -> PfqSetFilt/1
  Embedded MATLAB Function5/6(PfqRef) -> PfqRef/1
  Embedded MATLAB Function5/5(PrdSetFilt) -> PrdSetFilt/1
  Discrete-Time Integrator8/1 -> Embedded MATLAB Function5/5(x), x/1, Selector/1
  Id/1 -> Embedded MATLAB Function5/1(Id)
  Iq/1 -> Embedded MATLAB Function5/2(Iq)
  Embedded MATLAB Function5/1(Usd) -> Usd/1
  Tref/1 -> Embedded MATLAB Function5/3(Tref)
  Embedded MATLAB Function5/2(Usq) -> Usq/1
  Vbus/1 -> Embedded MATLAB Function5/4(Vbus)
  Embedded MATLAB Function5/4(PrdRef) -> PrdRef/1
  Embedded MATLAB Function5/8(wEst) -> wEst/1
  Embedded MATLAB Function5/9(PfdRef) -> PfdRef/1
  Selector1/1 -> ws/1
  Embedded MATLAB Function5/3(dx) -> Selector1/1, Discrete-Time Integrator8/1
  PrdSet/1 -> Embedded MATLAB Function5/6(PrdSet)

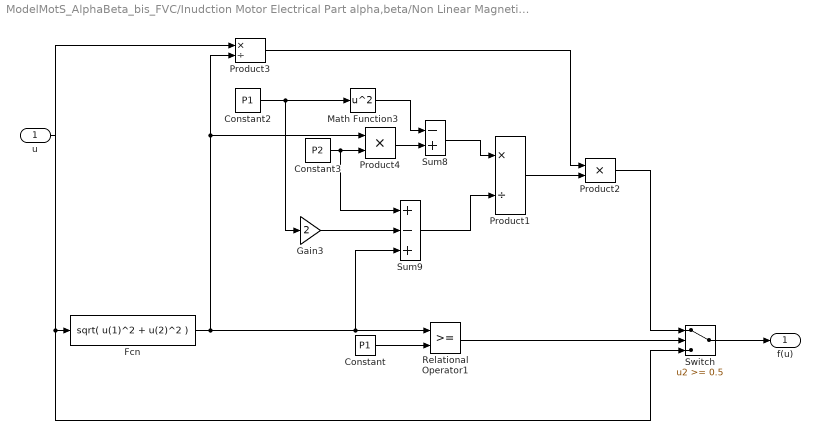
== system ModelMotS_AlphaBeta_bis_FVC/Inudction Motor Electrical Part alpha,beta/Non Linear Magnetic Coupling/f ==
  u : Inport
  Constant : Constant  Value=P1
  Constant2 : Constant  Value=P1
  Constant3 : Constant  Value=P2
  Fcn : Fcn  Expr=sqrt( u(1)^2 + u(2)^2 )
  Gain3 : Gain  Gain=2  SaturateOnIntegerOverflow=on  OutDataTypeStr=Inherit: Same as input  ParamDataTypeStr=Inherit: Same as input
  Math Function3 : Math  Operator=square  SaturateOnIntegerOverflow=on
  Product1 : Product  Inputs=*/  SaturateOnIntegerOverflow=on  RndMeth=Zero  InputSameDT=on  OutDataTypeStr=Inherit: Same as first input
  Product2 : Product  SaturateOnIntegerOverflow=on  RndMeth=Zero  InputSameDT=on  OutDataTypeStr=Inherit: Same as first input
  Product3 : Product  Inputs=*/  SaturateOnIntegerOverflow=on  RndMeth=Zero  InputSameDT=on  OutDataTypeStr=Inherit: Same as first input
  Product4 : Product  SaturateOnIntegerOverflow=on  RndMeth=Zero  InputSameDT=on  OutDataTypeStr=Inherit: Same as first input
  Relational Operator1 : RelationalOperator  RndMeth=Nearest  InputSameDT=on
  Sum8 : Sum  Inputs=-+  SaturateOnIntegerOverflow=on  InputSameDT=on  OutDataTypeStr=Inherit: Same as first input
  Sum9 : Sum  Inputs=+-+  SaturateOnIntegerOverflow=on  InputSameDT=on  OutDataTypeStr=Inherit: Same as first input
  Switch : Switch  Threshold=0.5  SaturateOnIntegerOverflow=on  InputSameDT=on
  f(u) : Outport  InitialOutput=0
  wires:
  Fcn/1 -> Sum9/3, Relational Operator1/1, Product4/1, Product3/2
  Switch/1 -> f(u)/1
  Sum8/1 -> Product1/1
  Sum9/1 -> Product1/2
  Constant2/1 -> Gain3/1, Math Function3/1
  Gain3/1 -> Sum9/2
  Constant3/1 -> Sum9/1, Product4/2
  Math Function3/1 -> Sum8/1
  Product4/1 -> Sum8/2
  Product1/1 -> Product2/2
  Product3/1 -> Product2/1
  u/1 -> Switch/3, Fcn/1, Product3/1
  Relational Operator1/1 -> Switch/2
  Constant/1 -> Relational Operator1/2
  Product2/1 -> Switch/1

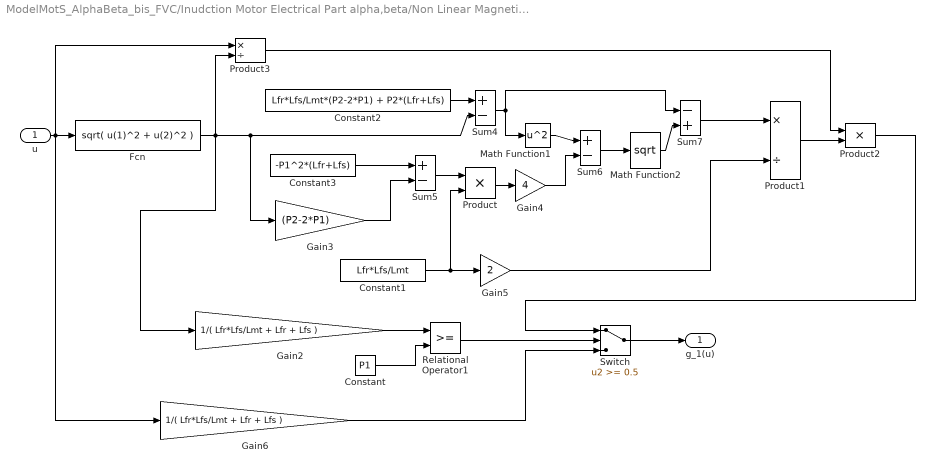
== system ModelMotS_AlphaBeta_bis_FVC/Inudction Motor Electrical Part alpha,beta/Non Linear Magnetic Coupling/g_1 ==
  u : Inport
  Constant : Constant  Value=P1
  Constant1 : Constant  Value=Lfr*Lfs/Lmt
  Constant2 : Constant  Value=Lfr*Lfs/Lmt*(P2-2*P1) + P2*(Lfr+Lfs)
  Constant3 : Constant  Value=-P1^2*(Lfr+Lfs)
  Fcn : Fcn  Expr=sqrt( u(1)^2 + u(2)^2 )
  Gain2 : Gain  Gain=1/( Lfr*Lfs/Lmt + Lfr + Lfs )  SaturateOnIntegerOverflow=on  OutDataTypeStr=Inherit: Same as input  ParamDataTypeStr=Inherit: Same as input
  Gain3 : Gain  Gain=(P2-2*P1)  SaturateOnIntegerOverflow=on  OutDataTypeStr=Inherit: Same as input  ParamDataTypeStr=Inherit: Same as input
  Gain4 : Gain  Gain=4  SaturateOnIntegerOverflow=on  OutDataTypeStr=Inherit: Same as input  ParamDataTypeStr=Inherit: Same as input
  Gain5 : Gain  Gain=2  SaturateOnIntegerOverflow=on  OutDataTypeStr=Inherit: Same as input  ParamDataTypeStr=Inherit: Same as input
  Gain6 : Gain  Gain=1/( Lfr*Lfs/Lmt + Lfr + Lfs )  SaturateOnIntegerOverflow=on  OutDataTypeStr=Inherit: Same as input  ParamDataTypeStr=Inherit: Same as input
  Math Function1 : Math  Operator=square  SaturateOnIntegerOverflow=on
  Math Function2 : Math  Operator=sqrt  SaturateOnIntegerOverflow=on
  Product : Product  SaturateOnIntegerOverflow=on  RndMeth=Zero  InputSameDT=on  OutDataTypeStr=Inherit: Same as first input
  Product1 : Product  Inputs=*/  SaturateOnIntegerOverflow=on  RndMeth=Zero  InputSameDT=on  OutDataTypeStr=Inherit: Same as first input
  Product2 : Product  SaturateOnIntegerOverflow=on  RndMeth=Zero  InputSameDT=on  OutDataTypeStr=Inherit: Same as first input
  Product3 : Product  Inputs=*/  SaturateOnIntegerOverflow=on  RndMeth=Zero  InputSameDT=on  OutDataTypeStr=Inherit: Same as first input
  Relational Operator1 : RelationalOperator  RndMeth=Nearest  InputSameDT=on
  Sum4 : Sum  Inputs=+-  SaturateOnIntegerOverflow=on  InputSameDT=on  OutDataTypeStr=Inherit: Same as first input
  Sum5 : Sum  Inputs=+-  SaturateOnIntegerOverflow=on  InputSameDT=on  OutDataTypeStr=Inherit: Same as first input
  Sum6 : Sum  Inputs=+-  SaturateOnIntegerOverflow=on  InputSameDT=on  OutDataTypeStr=Inherit: Same as first input
  Sum7 : Sum  Inputs=-+  SaturateOnIntegerOverflow=on  InputSameDT=on  OutDataTypeStr=Inherit: Same as first input
  Switch : Switch  Threshold=0.5  SaturateOnIntegerOverflow=on  InputSameDT=on
  g_1(u) : Outport  InitialOutput=0
  wires:
  Switch/1 -> g_1(u)/1
  Gain6/1 -> Switch/3
  Product2/1 -> Switch/1
  Constant/1 -> Relational Operator1/2
  Gain2/1 -> Relational Operator1/1
  Relational Operator1/1 -> Switch/2
  u/1 -> Gain6/1, Product3/1, Fcn/1
  Product3/1 -> Product2/1
  Fcn/1 -> Gain2/1, Product3/2, Gain3/1, Sum4/2
  Constant1/1 -> Gain5/1, Product/2
  Sum5/1 -> Product/1
  Product/1 -> Gain4/1
  Product1/1 -> Product2/2
  Gain5/1 -> Product1/2
  Sum7/1 -> Product1/1
  Gain3/1 -> Sum5/2
  Constant3/1 -> Sum5/1
  Sum4/1 -> Sum7/1, Math Function1/1
  Math Function2/1 -> Sum7/2
  Sum6/1 -> Math Function2/1
  Math Function1/1 -> Sum6/1
  Constant2/1 -> Sum4/1
  Gain4/1 -> Sum6/2

== matlab function ModelMotS_AlphaBeta_bis_FVC/Mechanical Part/Embedded MATLAB Function3 ==
  data: Tref output; dx output; wref input; wEst input; Tlim input; Kflux input; x input; wSpeed_PI parameter; xiSpeed_PI parameter; SFC_Coeff parameter; Jm parameter; np parameter
function [Tref, dx] = ControlLaw(wref, wEst,  Tlim, Kflux,x,wSpeed_PI,xiSpeed_PI,SFC_Coeff, Jm,np)
%#eml

%dx=[dwInputRef, dIsdSetFilt, dIsqSetFilt, ws, dwEst, dPfdE, dPfqE, dTint, dwd, dwq];


wInputRef=x(1);
Tint=x(2);

JmEst = Jm;

xi = xiSpeed_PI;
v0 = wSpeed_PI;
kp = JmEst/np*2*xi*v0;
ki = JmEst/np*v0^2; 

%%%%
%%%% Speed reference
%%%%                
   dwInputRef = ki/kp*( wref - wInputRef );   
   wInputRef2 = SFC_Coeff/100*wref + (1-SFC_Coeff/100)*wInputRef;
  
   wb = wEst;
   Tref = kp*(wInputRef2 - wb) + Tint;
   Trefbuf = Tref;
   if (abs(Tref)>Tlim) 
       Tref = sign(Tref)*Tlim; 
   end
   
   dTint = ( ki*(wInputRef2 - wb) + 1.5*ki/kp*(Tref - Trefbuf))*Kflux;
   
   dx=[dwInputRef, dTint];

== matlab function ModelMotS_AlphaBeta_bis_FVC/Electrical Part/Subsystem/Embedded MATLAB Function1 ==
  data: Kflux output; Tlim output; IsdFilt input; PfqSetFilt input; PfqRef input; PrdSetFilt input; PrdRef input; Rs parameter; Rr parameter; Ls parameter; Lr parameter; Lm parameter; Jm parameter; np parameter; Inom parameter; Prdnom parameter; Ilim input
function [Kflux, Tlim] = ControlLaw(IsdFilt,PfqSetFilt,PfqRef,PrdSetFilt,PrdRef, Rs,Rr,Ls,Lr,Lm,Jm,np,Inom, Prdnom,Ilim)
%#eml

Lf = Ls - Lm^2/Lr; 
Tr = Lr/Rr; 
invTr = 1/Tr; 
Rreq = Rr*(Lm/Lr)^2; 
Req = Rs + Rreq; 
L = Lm^2/Lr;
JmEst = Jm;
sig=Lf/Ls;

LfEst = Lf;
LEst = L;
invTrEst = invTr;
RsEst = Rs;
RreqEst = Rreq;
sigEst = sig;

%Ilim = 1.5*sqrt(2)*Inom;

PrdSet=Prdnom;
%%%%
%%%% Current Limitation
%%%%
   if (PrdSetFilt<PrdSet/64) Kflux = 1; 
   else if (PrdRef<PrdSet/64) Kflux = 1; 
   else Kflux = (PrdRef/PrdSetFilt)^2; 
   end;
   end;
   
   if (PrdSetFilt>PrdSet/16) 
     Tnorm = 3/2*np*PrdSetFilt*PrdSet/LEst;
   else
     Tnorm = 3/2*np*(PrdSet/16)*PrdSet/LEst;  
   end
   
   IdBC = IsdFilt;
   if ( (IdBC>Ilim) || (IdBC<-Ilim) )
       Tlim = 0.
   else 
       minU = 1;
       if ((PfqSetFilt*PrdRef*PrdSetFilt)~=0) minU = (PfqRef/PfqSetFilt)/(PrdRef/PrdSetFilt); end;
       if (minU > 2.) minU = 2.; else if (minU < 1.) minU = 1.; end; end; 
       IlimTMP = Ilim;
       IsqLim = sqrt(IlimTMP^2-IdBC^2)/minU;
       Tlim = 3/2*np*PrdRef*IsqLim/Kflux;
   end

== matlab function ModelMotS_AlphaBeta_bis_FVC/Electrical Part/Subsystem2/WsVdVq2/Embedded MATLAB Function5 ==
  data: Usd output; Usq output; Id input; dx output; Iq input; Tref input; Vbus input; x input; PrdSet input; Rs parameter; Rr parameter; Ls parameter; Lr parameter; Lm parameter; Jm parameter; np parameter; Vnom parameter; wCurr_PI parameter; xiCurr_PI parameter; Prdnom parameter; wCurr parameter; wSpeedEst parameter; PrdRef output; PrdSetFilt output; PfqRef output; PfqSetFilt output; wEst output; SLP_Coeff parameter; PfdRef output; Tpwm parameter; wMeas input
function [Usd, Usq, dx, PrdRef, PrdSetFilt, PfqRef, PfqSetFilt, wEst,PfdRef] = ControlLaw(Id,Iq,Tref,Vbus,x,PrdSet, Rs,Rr,Ls,Lr,Lm,Jm,np,Vnom,wCurr_PI,xiCurr_PI,Prdnom,wCurr,wSpeedEst,SLP_Coeff,Tpwm,wMeas)
%#eml

%   dx=[dIsdSetFilt, dIsqSetFilt, dPrdSetFilt, ws, dwEst, dPfdE, dPfqE, dPrdE, dwq];
IsdSetFilt=x(1);
IsqSetFilt=x(2);
PrdSetFilt=x(3);
PrqSetFilt=x(4);
Theta=x(5);
wEst=x(6);
PfdE=x(7);
PfqE=x(8);
PrdE=x(9);
PrqE=x(10);
wd=x(11);
wq=x(12);

Lf = Ls - Lm^2/Lr; 
Tr = Lr/Rr; 
invTr = 1/Tr; 
Rreq = Rr*(Lm/Lr)^2; 
Req = Rs + Rreq; 
L = Lm^2/Lr;
JmEst = Jm;
sig=Lf/Ls;

LfEst = Lf;
LEst = L;
invTrEst = invTr;
RsEst = Rs;
RreqEst = Rreq;
sigEst = sig;
ReqEst=RreqEst+RsEst;

vlim = Vbus/sqrt(3);

w1 = wCurr_PI;
w0 = 2*xiCurr_PI*w1;

PrdSet = Prdnom;
PfdSetFilt = LfEst*IsdSetFilt;
PfqSetFilt = LfEst*IsqSetFilt;
PfdRef = PfdE + PfdSetFilt;
PfqRef = PfqE + PfqSetFilt;
IsdRef = PfdRef/LfEst;
IsqRef = PfqRef/LfEst;
PrdRef = PrdE + PrdSetFilt ;
PrqRef = PrqE + PrqSetFilt ;

%%%%
%%%% Measure
%%%%

   IsdM = Id ;
   IsqM = Iq ;
   PfdM = LfEst*IsdM;
   PfqM = LfEst*IsqM;
   
%%%%
%%%% Set Point 
%%%%
   IPrdSet = PrdSet/LEst; 
   IsdSet = IPrdSet; 
   if (PrdSetFilt>PrdSet/16)
       IsqSet = (Tref/(3/2*np*PrdSetFilt));
   else
       IsqSet = (Tref/(3/2*np*PrdSet/16));
   end
   
   PfdSet = LfEst*IsdSet; 
   PfqSet = LfEst*IsqSet;

%%%%
%%%% Set Point Filtering
%%%%

    if (wCurr==0)
        wCurr1 = (RsEst+RreqEst)/LfEst;
    else
        wCurr1=wCurr;
    end
        
   dIsdSetFilt = wCurr1*(IsdSet - IsdSetFilt) ;
   dIsqSetFilt = wCurr1*(IsqSet - IsqSetFilt);

   Pfdq = PfdM + 1j*PfqM;
   PfdqRef = PfdRef + 1j*PfqRef; 
   PrdqRef = PrdRef + 1j*PrqRef;  
   IdqRef = PfdqRef/LfEst;

   wo = sqrt( invTrEst^2 + wEst^2 );
   lam = (RreqEst/LfEst)/wo;

   corVrE = (-RreqEst/LfEst-lam*(invTrEst+1j*wEst))*( - 0.);
   corVr = (-RreqEst/LfEst-lam*(invTrEst+1j*wEst))*(Pfdq-PfdqRef) ;
   
   dPrdSetFilt = invTrEst*(PrdSet-PrdSetFilt) - real(corVr);
   dPrqSetFilt = 0;

   PfdSetFilt = LfEst*IsdSetFilt; 
   PfqSetFilt = LfEst*IsqSetFilt;

%%%%
%%%% Stator Frequency
%%%%               
   if (PrdRef>PrdSet/16)
     wgCor= (RreqEst/LfEst*PfqRef -imag(corVr))/PrdRef;
   else
     wgCor= (RreqEst/LfEst*PfqRef -imag(corVr))/(PrdSet/16);  
   end
   
   dwEst = wSpeedEst*(wMeas - wEst);
   ws   = wEst + SLP_Coeff*wgCor/100.0 ;

%%%%
%%%% Gain Calculation
%%%%                   
   tempwd = (PfdRef-PfdM)/Prdnom;
   dwd = w1*w1*tempwd;
   propwd = w0*tempwd;   wdInt = propwd + wd;    
      
   tempwq = (PfqRef-PfqM)/Prdnom;
   dwq = w1*w1*tempwq;
   propwq = w0*tempwq;   wqInt = propwq + wq;           


%
% Voltage Calculation
%                
   UsdRef = (RsEst+RreqEst)/LfEst*PfdSetFilt + wCurr1*(PfdSet-PfdSetFilt) - ws*PfqSetFilt - invTrEst*PrdSetFilt + wdInt*Prdnom; 
   UsqRef = ws*PfdSetFilt + (RsEst+RreqEst)/LfEst*PfqSetFilt + wCurr1*(PfqSet-PfqSetFilt)+ wEst*PrdSetFilt + wqInt*Prdnom; 
   UsdqRef = sqrt( UsdRef^2+UsqRef^2);                   

%
% Voltage Limitation
%                
if (UsdqRef>vlim) 
   	Usd = UsdRef/UsdqRef*vlim; 
   	Usq = UsqRef/UsdqRef*vlim; 
else 
   Usd = UsdRef; Usq = UsqRef; 
end;

%
% FieldWeakening Calculation
%                
   
   Xd = Usd - UsdRef+ invTrEst*PrdE;
   Xq = Usq - UsqRef- wEst*PrdE; 
   Zd = (ReqEst/LfEst * Xd + ws * Xq)/(ReqEst^2/(LfEst*LfEst)+ws^2);
   Zq = (Req/LfEst * Xq - ws * Xd)/(ReqEst^2/(LfEst*LfEst)+ws^2);
   
   Bd = -PfdE + Zd;
   Bq = -PfqE + Zq;
   
   ThetaInc = ws*Tpwm;
   A11 = ((1-cos(ThetaInc))/Tpwm + cos(ThetaInc)*ReqEst/LfEst);
   A12 = (-sin(ThetaInc)/Tpwm + sin(ThetaInc)*ReqEst/LfEst);
   A21 = (sin(ThetaInc)/Tpwm - sin(ThetaInc)*ReqEst/LfEst);
   A22 = ((1-cos(ThetaInc))/Tpwm + cos(ThetaInc)*ReqEst/LfEst);
   
   dPfdE = A11*Bd + A12*Bq;
   dPfqE = A21*Bd + A22*Bq;
   
   dPrdE = (-invTrEst*PrdE + RreqEst/LfEst*PfdE );
   dPrqE = 0;   
   IsdE = PfdE/LfEst;
   IsqE = PfqE/LfEst;
   
   dx=[dIsdSetFilt; dIsqSetFilt; dPrdSetFilt,;dPrqSetFilt;, ws; dwEst; dPfdE; dPfqE; dPrdE;dPrqE; dwd; dwq];

== matlab function ModelMotS_AlphaBeta_bis_FVC/Electrical Part/Subsystem3/Embedded MATLAB Function2 ==
  data: Ia input; Id output; Ib input; theta input; Iq output
function [Id,Iq ] = RotCurrent(Ia,Ib,theta)
%#eml

Id = cos(theta)*Ia+sin(theta)*Ib;
Iq = -sin(theta)*Ia+cos(theta)*Ib;

== matlab function ModelMotS_AlphaBeta_bis_FVC/Electrical Part/Subsystem1/Embedded MATLAB Function5 ==
  data: Vd input; Va output; Vq input; theta input; Vb output; thetaInc input
function [Va,Vb ] = RotVoltage(Vd,Vq,theta, thetaInc)
%#eml

if (thetaInc~=0)
    ktheta=sin(thetaInc/2)/(thetaInc/2);
else
    ktheta=1;
end

Vdloc=ktheta*Vd;
Vqloc=ktheta*Vq;

Va = cos(theta+thetaInc/2)*Vdloc-sin(theta+thetaInc/2)*Vqloc;
Vb = sin(theta+thetaInc/2)*Vdloc+cos(theta+thetaInc/2)*Vqloc;
% 
% V1 = Va;
% V2 = -1/2*Va+sqrt(3)/2*Vb;
% V3 = -1/2*Va-sqrt(3)/2*Vb;
